simulink model "Memoria"  (R2023b)
settings: Solver=VariableStepAuto  StartTime=0.0  StopTime=5  RelTol=1e-3
settings Model: Creator=Alejandro Villeda  LastModifiedBy=diavl

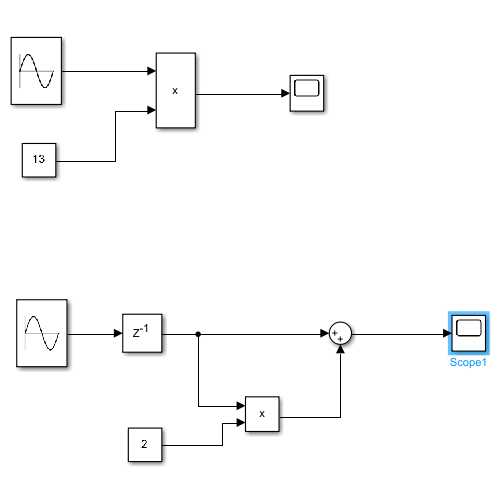
[thumbnail: Simulink's stored preview of the top-level diagram]
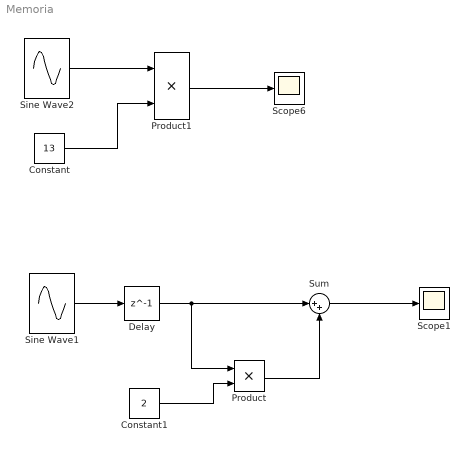
== system Memoria ==
  Constant : Constant  Value=13
  Constant1 : Constant  Value=2
  Delay : Delay  DelayLength=1  InitialCondition=0  SampleTime=50e-6
  Product : Product
  Product1 : Product
  Scope1 : Scope
  Scope6 : Scope
  Sine Wave1 : Sin  Frequency=pi  SampleTime=0
  Sine Wave2 : Sin  Frequency=pi  SampleTime=0
  Sum : Sum  Inputs=|++
  wires:
  Product1/1 -> Scope6/1
  Sine Wave2/1 -> Product1/1
  Constant/1 -> Product1/2
  Sum/1 -> Scope1/1
  Sine Wave1/1 -> Delay/1
  Delay/1 -> Sum/1, Product/1
  Constant1/1 -> Product/2
  Product/1 -> Sum/2
